simulink model "L5"  (R2023a)
settings: Solver=VariableStepAuto  StartTime=0.0  StopTime=1  RelTol=1e-8
undefined symbols (not defined in the file): K, T
settings Model: Creator=apere  LastModifiedBy=apere

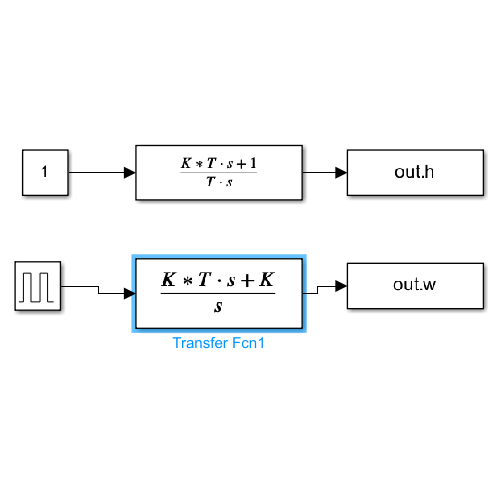
[thumbnail: Simulink's stored preview of the top-level diagram]
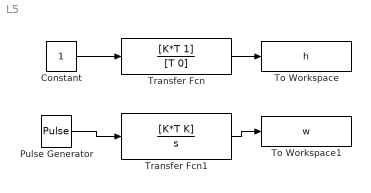
== system L5 ==
  Constant : Constant
  Pulse Generator : DiscretePulseGenerator  PulseType=Time based  Period=10  PulseWidth=5
  To Workspace : ToWorkspace  VariableName=h  SaveFormat=Timeseries  SampleTime=-1
  To Workspace1 : ToWorkspace  VariableName=w  SaveFormat=Timeseries  SampleTime=-1
  Transfer Fcn : TransferFcn  Numerator=[K*T 1]  Denominator=[T 0]
  Transfer Fcn1 : TransferFcn  Numerator=[K*T K]  Denominator=[1 0]
  wires:
  Constant/1 -> Transfer Fcn/1
  Transfer Fcn/1 -> To Workspace/1
  Pulse Generator/1 -> Transfer Fcn1/1
  Transfer Fcn1/1 -> To Workspace1/1
